simulink model "parallel_clipper"  (R2015a)
settings: Solver=ode45  StartTime=0.0  StopTime=0.05  RelTol=1e-3
libraries: powerlib x7
settings Model: Creator=asus  LastModifiedBy=asus

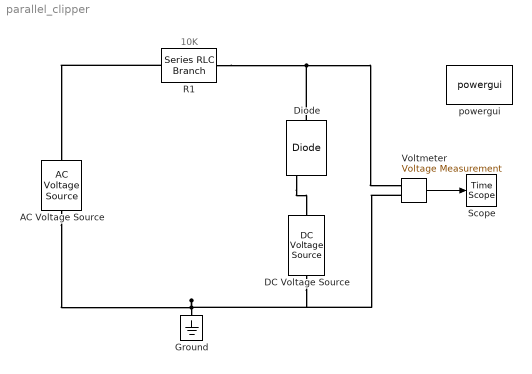
== system parallel_clipper ==
  note: 10K
  AC Voltage Source : powerlib/Electrical Sources/AC Voltage Source  Amplitude=12  Phase=0  Frequency=60  SampleTime=0  Measurements=Voltage
  DC Voltage Source : powerlib/Electrical Sources/DC Voltage Source  Amplitude=4  Measurements=Voltage
  Diode : powerlib/Power Electronics/Diode  Ron=0.001  Lon=0  Vf=0.8  IC=0  UseSnubber=off  Rs=0  Cs=0  Measurements=on
  Ground : powerlib/Elements/Ground  LConnTagsString=a
  R1 : powerlib/Elements/Series RLC Branch  LConnTagsString=__new0  RConnTagsString=__new0  BranchType=R  Resistance=1000  Inductance=1e-3  SetiL0=off  InitialCurrent=0  Capacitance=1e-6  Setx0=off  InitialVoltage=0  Measurements=None
  Scope : TimeScope
  Voltmeter : powerlib/Measurements/Voltage Measurement  PhasorSimulation=off  OutputType=Complex  PSBequivalent=0
  powergui : powerlib/powergui  Priority=1  SimulationMode=Discrete  SolverType=Tustin/Backward Euler (TBE)  SampleTime=10e-6  frequency=60  SPID=off  DisableSnubberDevices=off  DisableRonSwitches=off  DisableVfSwitches=off  SwTol=0  DisplayEquations=off  Interpol=off  methode=off  Ts=100  FunctionMessages=off  echomessages=off  HookPort=off  EnableUseOfTLC=off  x0status=blocks  frequencyindice=0  Pbase=100e6  ErrMax=1e-4  Iterations=50  UnitsV=kV  UnitsW=MW  buscounter=0  RestoreLinks=warning  ResistiveCurrentMeasurement=off  Frange=[0:2:500]  Ylog=off  Xlog=on  ShowGrid=off  save=off  variable=ZData  structure=0  ZoomFFT=off  StartTime=0.0  cycles=1  DisplayStyle=1  fundamental=60  FreqAxis=off  MaxFrequency=1000  frequencyindicesteady=1  RmsSteady=1  display=off
  wires:
  Voltmeter/1 -> Scope/1
  connections:
  Ground/LConn1 -- DC Voltage Source/LConn1 -- Voltmeter/LConn2 -- AC Voltage Source/LConn1
  R1/RConn1 -- Diode/LConn1 -- Voltmeter/LConn1
  R1/LConn1 -- AC Voltage Source/RConn1
  Diode/RConn1 -- DC Voltage Source/RConn1
